simulink model "debugTxSync"  (R2024a)
settings: Solver=FixedStepDiscrete  StartTime=0.0  StopTime=10.0  RelTol=1e-3
libraries: simulink x2, hdlsllib x2
settings Model: DataTypeOverride=Off  Creator=cotti  LastModifiedBy=cotti
settings OptimizationCC: BlockReduction=off  ConditionallyExecuteInputs=off  DefaultParameterBehavior=Inlined  InheritOutputTypeSmallerThanSingle=on
settings DebuggingCC: AlgebraicLoopMsg=error  ArtificialAlgebraicLoopMsg=error  SingleTaskRateTransMsg=error  UnconnectedInputMsg=warning  UnconnectedOutputMsg=warning  UnconnectedLineMsg=warning
settings HardwareCC: ProdBitPerPointer=32  ProdBitPerSizeT=32  ProdBitPerPtrDiffT=32  ProdLargestAtomicFloat=None  ProdIntDivRoundTo=Undefined  ProdEndianess=Unspecified  ProdWordSize=32  ProdHWDeviceType=ASIC/FPGA->ASIC/FPGA  TargetBitPerLong=64  TargetBitPerPointer=64  TargetBitPerSizeT=64  TargetBitPerPtrDiffT=64  TargetLongLongMode=on  TargetIntDivRoundTo=Zero  TargetEndianess=LittleEndian  TargetWordSize=64  TargetHWDeviceType=Custom Processor->MATLAB Host Computer  ProdEqTarget=off

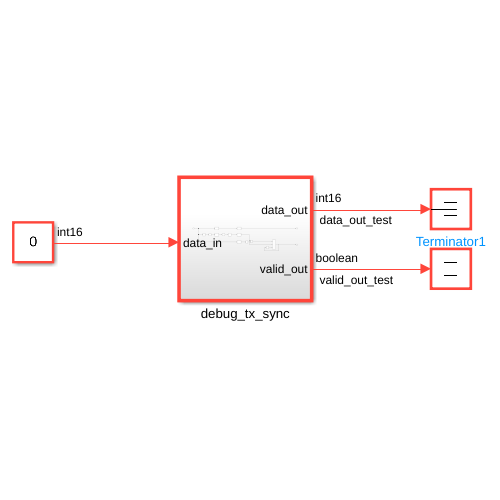
[thumbnail: Simulink's stored preview of the top-level diagram]
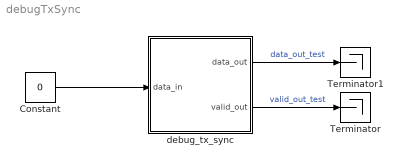
== system debugTxSync ==
  Constant : Constant  Value=0  OutDataTypeStr=int16  SampleTime=-1
  Terminator : Terminator
  Terminator1 : Terminator
  debug_tx_sync : Subsystem  TreatAsAtomicUnit=on
  wires:
  debug_tx_sync/2(valid_out) -> Terminator/1  "valid_out_test"
  debug_tx_sync/1(data_out) -> Terminator1/1  "data_out_test"
  Constant/1 -> debug_tx_sync/1(data_in)

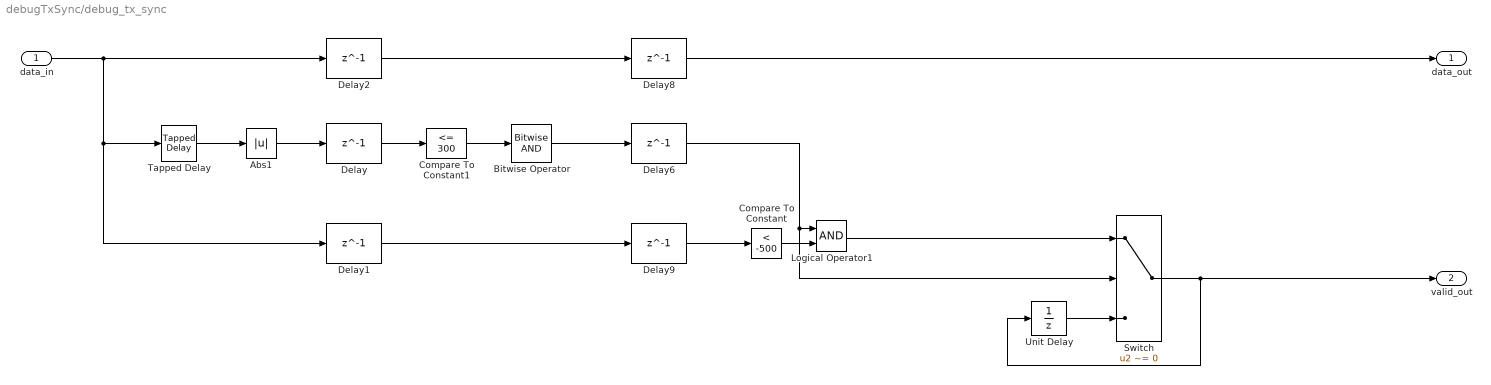
== system debugTxSync/debug_tx_sync ==
  data_in : Inport
  Abs1 : Abs  SaturateOnIntegerOverflow=off
  Bitwise Operator : simulink/Logic and Bit Operations/Bitwise Operator  logicop=AND  UseBitMask=off  BitMask=bin2dec('11011001')  BitMaskRealWorld=Stored Integer
      settings: LibrarySourceBlock=|
      | hdlsllib/Logic and Bit
      | Operations/Bitwise
      | Operator
  Compare To Constant : hdlsllib/Logic and Bit Operations/Compare To Constant  relop=<  const=-500  OutDataTypeStr=boolean
  Compare To Constant1 : hdlsllib/Logic and Bit Operations/Compare To Constant  relop=<=  const=300  OutDataTypeStr=boolean
  Delay{,1..2,6,8..9} (6 alike) : Delay  DelayLength=1  InitialCondition=0  UseCircularBuffer=on
  Logical Operator1 : Logic  AllPortsSameDT=off  OutDataTypeStr=boolean
  Switch : Switch  Criteria=u2 ~= 0  SaturateOnIntegerOverflow=off  InputSameDT=off
  Tapped Delay : simulink/Discrete/Tapped Delay  vinit=0.0  samptime=-1  NumDelays=8  DelayOrder=Oldest  includeCurrent=off
      settings: LibrarySourceBlock=hdlsllib/Discrete/Tapped Delay
  Unit Delay : UnitDelay  SampleTime=-1  HasFrameUpgradeWarning=on
  data_out : Outport
  valid_out : Outport  Port=2
  wires:
  Tapped Delay/1 -> Abs1/1
  Abs1/1 -> Delay/1
  Switch/1 -> Unit Delay/1, valid_out/1
  Delay/1 -> Compare To Constant1/1
  Logical Operator1/1 -> Switch/1
  Unit Delay/1 -> Switch/3
  Bitwise Operator/1 -> Delay6/1
  data_in/1 -> Delay2/1, Delay1/1, Tapped Delay/1
  Compare To Constant/1 -> Logical Operator1/2
  Compare To Constant1/1 -> Bitwise Operator/1
  Delay1/1 -> Delay9/1
  Delay2/1 -> Delay8/1
  Delay6/1 -> Switch/2, Logical Operator1/1
  Delay8/1 -> data_out/1
  Delay9/1 -> Compare To Constant/1
